simulink model "SteadyStateAccelerationModel"  (R2018a)
settings: Solver=VariableStepAuto  StartTime=0.0  StopTime=25  FixedStep=1e-3  MaxStep=1e-2  RelTol=1e-5
PreLoadFcn:
  | modelDir = fileparts(get_param(bdroot, 'FileName'));
  | addpath(fullfile(modelDir,'../../Parameters'));
  | addpath(fullfile(modelDir,'../../Model/generated'));
  | addpath(fullfile(modelDir,'../../Misc'));
  | 
  | Parameters_Simulation
  | Constants_Kugle
  | Constants_nominal
InitFcn:
  | Parameters_Simulation
  | Constants_Kugle
  | Constants_nominal
undefined symbols (not defined in the file or in its folder): COM, constants, x_init
settings Model: Creator=Thomas  LastModifiedBy=Thomas
settings DataIOCC: SaveOutput=off  SignalLogging=off  DSMLogging=off
settings DebuggingCC: UniqueDataStoreMsg=error
settings HardwareCC: ProdBitPerPointer=32  ProdBitPerSizeT=32  ProdBitPerPtrDiffT=32  ProdLargestAtomicInteger=Long  ProdLargestAtomicFloat=Double  ProdWordSize=32  ProdHWDeviceType=ARM Compatible->ARM Cortex
settings ModelReferenceCC: ModelReferenceMinAlgLoopOccurrences=on
settings RTWCC: GenCodeOnly=on  Toolchain=GNU Tools for ARM Embedded Processors
settings GRTTargetCC: TargetLangStandard=C89/C90 (ANSI)  CodeReplacementLibrary=ARM Cortex-M (CMSIS)

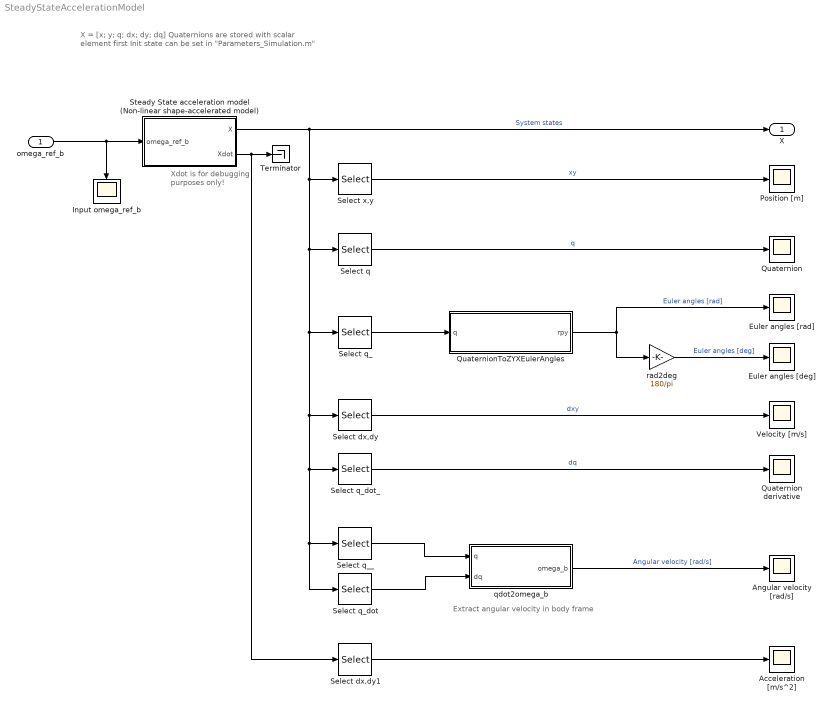
== system SteadyStateAccelerationModel ==
  note: X = [x; y; q; dx; dy; dq]
      | Quaternions are stored with scalar element first
      | Init state can be set in "Parameters_Simulation.m"
  note: Extract angular velocity in body frame
  note: Xdot is for debugging
      | purposes only!
  omega_ref_b : Inport  PortDimensions=3
  Acceleration [m/s^2] : Scope
  Angular velocity [rad/s] : Scope
  Euler angles [deg] : Scope
  Euler angles [rad] : Scope
  Input omega_ref_b : Scope
  Position [m] : Scope
  Quaternion : Scope
  Quaternion derivative : Scope
  QuaternionToZYXEulerAngles : MATLAB Function  TreatAsAtomicUnit=on
  Select dx,dy : Selector  InputPortWidth=12  IndexOptions=Index vector (dialog)  Indices=[7,8]  OutputSizes=1
  Select dx,dy1 : Selector  InputPortWidth=12  IndexOptions=Index vector (dialog)  Indices=[7,8]  OutputSizes=1
  Select q : Selector  InputPortWidth=12  IndexOptions=Index vector (dialog)  Indices=[3,4,5,6]  OutputSizes=1
  Select q_ : Selector  InputPortWidth=12  IndexOptions=Index vector (dialog)  Indices=[3,4,5,6]  OutputSizes=1
  Select q__ : Selector  InputPortWidth=12  IndexOptions=Index vector (dialog)  Indices=[3,4,5,6]  OutputSizes=1
  Select q_dot : Selector  InputPortWidth=12  IndexOptions=Index vector (dialog)  Indices=[9,10,11,12]  OutputSizes=1
  Select q_dot_ : Selector  InputPortWidth=12  IndexOptions=Index vector (dialog)  Indices=[9,10,11,12]  OutputSizes=1
  Select x,y : Selector  InputPortWidth=12  IndexOptions=Index vector (dialog)  Indices=[1,2]  OutputSizes=1
  Steady State acceleration model (Non-linear shape-accelerated model) : Subsystem
  Terminator : Terminator
  Velocity [m/s] : Scope
  qdot2omega_b : MATLAB Function  TreatAsAtomicUnit=on
  rad2deg : Gain  Gain=180/pi
  X : Outport
  wires:
  Select dx,dy1/1 -> Acceleration [m/s^2]/1
  Select q__/1 -> qdot2omega_b/1(q)
  rad2deg/1 -> Euler angles [deg]/1  "Euler angles [deg]"
  QuaternionToZYXEulerAngles/1(rpy) -> rad2deg/1, Euler angles [rad]/1  "Euler angles [rad]"
  Steady State acceleration model (Non-linear shape-accelerated model)/2(Xdot) -> Terminator/1, Select dx,dy1/1
  Select dx,dy/1 -> Velocity [m/s]/1  "dxy"
  Select q_dot_/1 -> Quaternion derivative/1  "dq"
  Select q/1 -> Quaternion/1  "q"
  qdot2omega_b/1(omega_b) -> Angular velocity [rad/s]/1  "Angular velocity [rad/s]"
  Steady State acceleration model (Non-linear shape-accelerated model)/1(X) -> Select x,y/1, Select q__/1, Select q_dot/1, Select q_dot_/1, Select dx,dy/1, Select q_/1, Select q/1, X/1  "System states"
  Select x,y/1 -> Position [m]/1  "xy"
  Select q_dot/1 -> qdot2omega_b/2(dq)
  Select q_/1 -> QuaternionToZYXEulerAngles/1(q)
  omega_ref_b/1 -> Input omega_ref_b/1, Steady State acceleration model (Non-linear shape-accelerated model)/1(omega_ref_b)

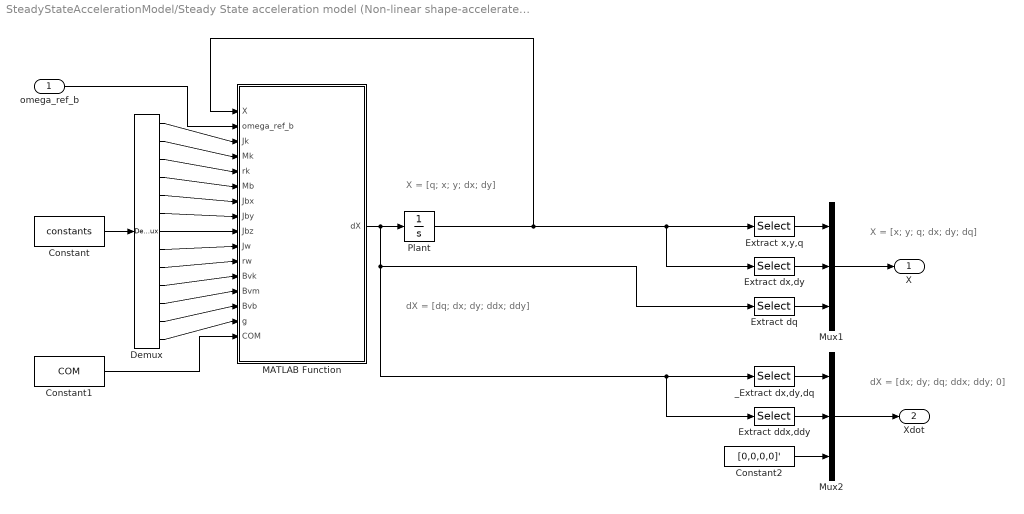
== system SteadyStateAccelerationModel/Steady State acceleration model (Non-linear shape-accelerated model) ==
  note: X = [x; y; q; dx; dy; dq]
  note: X = [q; x; y; dx; dy]
  note: dX = [dq; dx; dy; ddx; ddy]
  note: dX = [dx; dy; dq; ddx; ddy; 0]
  omega_ref_b : Inport
  Constant : Constant  Value=constants
  Constant1 : Constant  Value=COM
  Constant2 : Constant  Value=[0,0,0,0]'
  Demux : Demux  Outputs=13
  Extract ddx,ddy : Selector  InputPortWidth=8  IndexOptions=Index vector (dialog)  Indices=[7 8]  OutputSizes=1
  Extract dq : Selector  InputPortWidth=8  IndexOptions=Index vector (dialog)  Indices=[1 2 3 4]  OutputSizes=1
  Extract dx,dy : Selector  InputPortWidth=8  IndexOptions=Index vector (dialog)  Indices=[7 8]  OutputSizes=1
  Extract x,y,q : Selector  InputPortWidth=8  IndexOptions=Index vector (dialog)  Indices=[5 6 1 2 3 4]  OutputSizes=1
  MATLAB Function : MATLAB Function  TreatAsAtomicUnit=on
  Mux1 : Mux  Inputs=3
  Mux2 : Mux  Inputs=3
  Plant : Integrator  InitialCondition=[x_init(3:6); x_init(1:2); x_init(7:8)]
  _Extract dx,dy,dq : Selector  InputPortWidth=8  IndexOptions=Index vector (dialog)  Indices=[5 6 1 2 3 4]  OutputSizes=1
  X : Outport
  Xdot : Outport  Port=2
  wires:
  Demux/12 -> MATLAB Function/14(Bvb)
  Demux/11 -> MATLAB Function/13(Bvm)
  Demux/5 -> MATLAB Function/7(Jbx)
  Demux/8 -> MATLAB Function/10(Jw)
  Demux/1 -> MATLAB Function/3(Jk)
  Constant/1 -> Demux/1
  Demux/3 -> MATLAB Function/5(rk)
  Demux/6 -> MATLAB Function/8(Jby)
  Demux/7 -> MATLAB Function/9(Jbz)
  Demux/10 -> MATLAB Function/12(Bvk)
  Demux/2 -> MATLAB Function/4(Mk)
  Demux/9 -> MATLAB Function/11(rw)
  Demux/4 -> MATLAB Function/6(Mb)
  omega_ref_b/1 -> MATLAB Function/2(omega_ref_b)
  Plant/1 -> Extract dx,dy/1, Extract x,y,q/1, MATLAB Function/1(X)
  Constant1/1 -> MATLAB Function/16(COM)
  Demux/13 -> MATLAB Function/15(g)
  Extract x,y,q/1 -> Mux1/1
  Mux1/1 -> X/1
  MATLAB Function/1(dX) -> Extract ddx,ddy/1, _Extract dx,dy,dq/1, Extract dq/1, Plant/1
  Mux2/1 -> Xdot/1
  _Extract dx,dy,dq/1 -> Mux2/1
  Extract dx,dy/1 -> Mux1/2
  Extract dq/1 -> Mux1/3
  Extract ddx,ddy/1 -> Mux2/2
  Constant2/1 -> Mux2/3

== matlab function SteadyStateAccelerationModel/QuaternionToZYXEulerAngles ==
  data: q input; rpy output
function rpy = Quaternion2ZYXEulerAngles(q)
    rpy = Quaternion2ZYXEulerAngles(q);
end

== matlab function SteadyStateAccelerationModel/Steady State acceleration model (Non-linear shape-accelerated model)/MATLAB Function ==
  data: dX output size=8; X input size=8; omega_ref_b input size=3; Jk input; Mk input; rk input; Mb input; Jbx input; Jby input; Jbz input; Jw input; rw input; Bvk input; Bvm input; Bvb input; g input; COM input size=3
function dX = NonlinearMPCmodel(X,omega_ref_b,Jk,Mk,rk,Mb,Jbx,Jby,Jbz,Jw,rw,Bvk,Bvm,Bvb,g,COM)
    Phi = @(q)[q(1) -q(2) -q(3) -q(4);     % for q o p = Phi(q) * p
              q(2) q(1)  -q(4) q(3);
              q(3) q(4)  q(1)  -q(2);
              q(4) -q(3) q(2)  q(1)];           
    Gamma = @(p)[p(1) -p(2) -p(3) -p(4);   % for q o p = Gamma(p) * q
                 p(2) p(1) p(4) -p(3);
                 p(3) -p(4) p(1) p(2);
                 p(4) p(3) -p(2) p(1)];  

    devec = [0,1,0,0;0,0,1,0;0,0,0,1]; % 'v' in notes
    vec = [0,0,0;1,0,0;0,1,0;0,0,1]; % '^' in notes
    I_conj = diag([1,-1,-1,-1]);    

    COM_X = COM(1);
    COM_Y = COM(2);
    COM_Z = COM(3);
    
    % Extract states
    q1 = X(1);
    q2 = X(2);
    q3 = X(3);
    q4 = X(4);
    x = X(5);
    y = X(6);
    dx = X(7);
    dy = X(8);
    
    q = [q1,q2,q3,q4]';   
    
    % Non-linear ODE/model equations    
    %dq = 1/2 * Gamma(q) * vec * omega_ref; % inertial frame omega_ref
    dq = 1/2 * Phi(q) * vec * omega_ref_b; % body frame omega_ref    
        
    acceleration = SteadyStateAcceleration(COM_X,COM_Y,COM_Z,Jk,Jw,Mb,Mk,dx,dy,g,q1,q2,q3,q4,rk,rw);    
    ddx = acceleration(1);
    ddy = acceleration(2);
    
    dX = [dq; dx; dy; ddx; ddy];

== matlab function SteadyStateAccelerationModel/qdot2omega_b ==
  data: q input; omega_b output; dq input
function omega_b = qdot2omega_b(q, dq)
    omega_b = qdot2omega_b(q, dq);
end
